simulink model "Project1_1"  (R2017a)
settings: Solver=ode45  StartTime=0.0  StopTime=0.5  MaxStep=1e-4  RelTol=1e-3
settings Model: Creator=Callum  LastModifiedBy=Callum

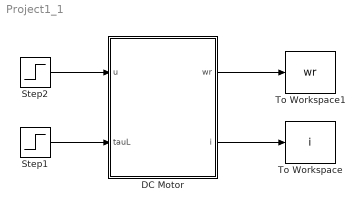
== system Project1_1 ==
  DC Motor : Subsystem  mask{R=0.5, L=2.5e-3, psi=0.35, J=1e-3}
      mask prompts: R "R (ohm)"; L "L (H)"; psi "psi(Vs)"; J "J (kgm^2)"
  Step1 : Step  Time=0.3  After=7  SampleTime=0
  Step2 : Step  Time=0.1  After=120  SampleTime=0
  To Workspace : ToWorkspace  VariableName=i  SaveFormat=Timeseries  SampleTime=-1
      settings: Save2DSignal=2-D array (concatenate along first dimension)
  To Workspace1 : ToWorkspace  VariableName=wr  SaveFormat=Timeseries  SampleTime=-1
      settings: Save2DSignal=2-D array (concatenate along first dimension)
  wires:
  DC Motor/2(i) -> To Workspace/1
  DC Motor/1(wr) -> To Workspace1/1
  Step1/1 -> DC Motor/2(tauL)
  Step2/1 -> DC Motor/1(u)

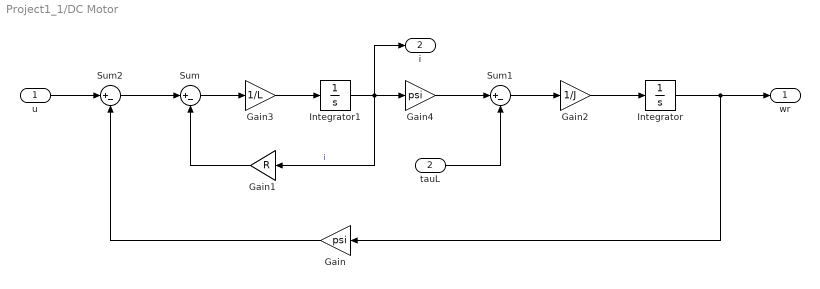
== system Project1_1/DC Motor ==
  u : Inport
  tauL : Inport  Port=2
  Gain : Gain  Gain=psi
  Gain1 : Gain  Gain=R
  Gain2 : Gain  Gain=1/J
  Gain3 : Gain  Gain=1/L
  Gain4 : Gain  Gain=psi
  Integrator : Integrator
  Integrator1 : Integrator
  Sum : Sum  Inputs=|+-
  Sum1 : Sum  Inputs=|+-
  Sum2 : Sum  Inputs=|+-
  wr : Outport
  i : Outport  Port=2
  wires:
  u/1 -> Sum2/1
  Integrator1/1 -> i/1, Gain1/1, Gain4/1  "i"
  Gain/1 -> Sum2/2
  tauL/1 -> Sum1/2
  Gain4/1 -> Sum1/1
  Integrator/1 -> wr/1, Gain/1
  Sum1/1 -> Gain2/1
  Gain2/1 -> Integrator/1
  Sum/1 -> Gain3/1
  Sum2/1 -> Sum/1
  Gain3/1 -> Integrator1/1
  Gain1/1 -> Sum/2
